simulink subsystem "RoboRio_Controls_sub"  (R2023b)
settings: Solver=VariableStepAuto  StartTime=0.0  StopTime=10.0  RelTol=1e-3
undefined symbols (not defined in the file): Climber_DutyCycle_Neg, Climber_DutyCycle_Pos, Odometry_IC_X, Odometry_IC_Y
libraries: simulink x3, Autonomous_lib x1, Disabled_lib x1, Teleop_lib x1, Test_lib x1
(part 2 of 2)

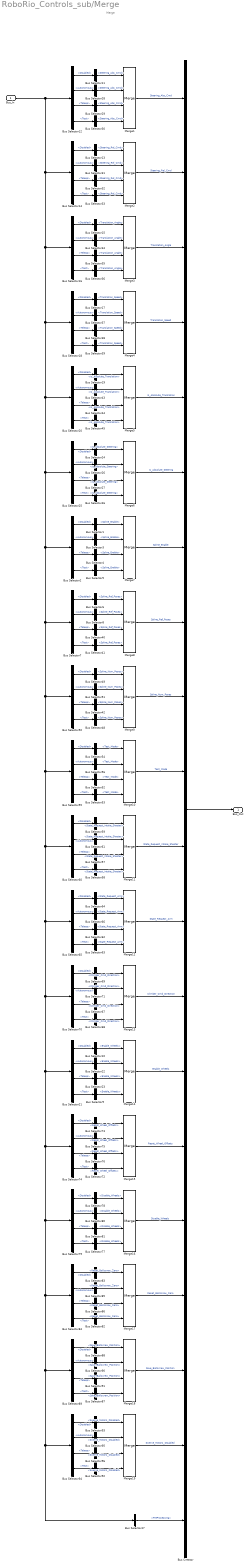
== system RoboRio_Controls_sub/Merge ==
  note: Merge
  Bus_In : Inport
  Bus Creator : BusCreator  Inputs=20
  Bus Selector{1,3..5} (4 alike) : BusSelector  OutputSignals=Spline_Enable
  Bus Selector{9..10,22..23} (4 alike) : BusSelector  OutputSignals=Enable_Wheels
  Bus Selector{11,28..30} (4 alike) : BusSelector  OutputSignals=Steering_Abs_Cmd
  Bus Selector{2,7,12,14,16,18,20..21,25,50,55,60,65,70,74,79,84,89,94} (19 alike) : BusSelector  OutputSignals=Disabled,Autonomous,Teleop,Test
  Bus Selector{13,31..33} (4 alike) : BusSelector  OutputSignals=Steering_Rel_Cmd
  Bus Selector{15,34..36} (4 alike) : BusSelector  OutputSignals=Translation_Angle
  Bus Selector{17,37..39} (4 alike) : BusSelector  OutputSignals=Translation_Speed
  Bus Selector{19,43..45} (4 alike) : BusSelector  OutputSignals=Is_Absolute_Translation
  Bus Selector{24,26..27,46} (4 alike) : BusSelector  OutputSignals=Is_Absolute_Steering
  Bus Selector{6,8,40..41} (4 alike) : BusSelector  OutputSignals=Spline_Ref_Poses
  Bus Selector{42,48..49,51} (4 alike) : BusSelector  OutputSignals=Spline_Num_Poses
  Bus Selector47 : BusSelector  OutputSignals=PreProcessing
  Bus Selector{52..54,56} (4 alike) : BusSelector  OutputSignals=Test_Mode
  Bus Selector{57..59,61} (4 alike) : BusSelector  OutputSignals=State_Request_Intake_Shooter
  Bus Selector{62..64,66} (4 alike) : BusSelector  OutputSignals=State_Request_Arm
  Bus Selector{67..69,71} (4 alike) : BusSelector  OutputSignals=Climber_Cmd_Direction
  Bus Selector{72..73,75..76} (4 alike) : BusSelector  OutputSignals=Reset_Wheel_Offsets
  Bus Selector{77..78,80..81} (4 alike) : BusSelector  OutputSignals=Disable_Wheels
  Bus Selector{82..83,85..86} (4 alike) : BusSelector  OutputSignals=Reset_Ballscrew_Zero
  Bus Selector{87..88,90..91} (4 alike) : BusSelector  OutputSignals=Save_Ballscrew_Position
  Bus Selector{92..93,95..96} (4 alike) : BusSelector  OutputSignals=Swerve_Motors_Disabled
  Merge{1..19} (19 alike) : Merge  Inputs=4
  Bus_Out : Outport
  wires:
  Bus Creator/1 -> Bus_Out/1
  Merge14/1 -> Bus Creator/14  "Enable_Wheels"
  Bus Selector21/4 -> Bus Selector9/1  "<Test>"
  Bus Selector9/1 -> Merge14/4  "<Enable_Wheels>"
  Bus Selector21/3 -> Bus Selector23/1  "<Teleop>"
  Bus Selector21/2 -> Bus Selector22/1  "<Autonomous>"
  Bus Selector10/1 -> Merge14/1  "<Enable_Wheels>"
  Bus_In/1 -> Bus Selector12/1, Bus Selector14/1, Bus Selector16/1, Bus Selector18/1, Bus Selector20/1, Bus Selector25/1, Bus Selector60/1, Bus Selector21/1, Bus Selector74/1, Bus Selector79/1, Bus Selector84/1, Bus Selector89/1, Bus Selector94/1, Bus Selector47/1, Bus Selector70/1, Bus Selector65/1, Bus Selector55/1, Bus Selector50/1, Bus Selector7/1, Bus Selector2/1
  Bus Selector22/1 -> Merge14/2  "<Enable_Wheels>"
  Bus Selector21/1 -> Bus Selector10/1  "<Disabled>"
  Bus Selector23/1 -> Merge14/3  "<Enable_Wheels>"
  Bus Selector94/4 -> Bus Selector92/1  "<Test>"
  Bus Selector93/1 -> Merge19/1  "<Swerve_Motors_Disabled>"
  Bus Selector94/2 -> Bus Selector95/1  "<Autonomous>"
  Bus Selector92/1 -> Merge19/4  "<Swerve_Motors_Disabled>"
  Bus Selector94/3 -> Bus Selector96/1  "<Teleop>"
  Bus Selector94/1 -> Bus Selector93/1  "<Disabled>"
  Bus Selector96/1 -> Merge19/3  "<Swerve_Motors_Disabled>"
  Bus Selector95/1 -> Merge19/2  "<Swerve_Motors_Disabled>"
  Merge19/1 -> Bus Creator/19  "Swerve_Motors_Disabled"
  Merge18/1 -> Bus Creator/18  "Save_Ballscrew_Position"
  Bus Selector89/4 -> Bus Selector87/1  "<Test>"
  Bus Selector88/1 -> Merge18/1  "<Save_Ballscrew_Position>"
  Bus Selector91/1 -> Merge18/3  "<Save_Ballscrew_Position>"
  Bus Selector89/3 -> Bus Selector91/1  "<Teleop>"
  Bus Selector89/2 -> Bus Selector90/1  "<Autonomous>"
  Bus Selector89/1 -> Bus Selector88/1  "<Disabled>"
  Bus Selector87/1 -> Merge18/4  "<Save_Ballscrew_Position>"
  Bus Selector90/1 -> Merge18/2  "<Save_Ballscrew_Position>"
  Bus Selector84/3 -> Bus Selector86/1  "<Teleop>"
  Bus Selector85/1 -> Merge17/2  "<Reset_Ballscrew_Zero>"
  Merge17/1 -> Bus Creator/17  "Reset_Ballscrew_Zero"
  Bus Selector82/1 -> Merge17/4  "<Reset_Ballscrew_Zero>"
  Bus Selector84/4 -> Bus Selector82/1  "<Test>"
  Bus Selector84/2 -> Bus Selector85/1  "<Autonomous>"
  Bus Selector83/1 -> Merge17/1  "<Reset_Ballscrew_Zero>"
  Bus Selector86/1 -> Merge17/3  "<Reset_Ballscrew_Zero>"
  Bus Selector84/1 -> Bus Selector83/1  "<Disabled>"
  Merge16/1 -> Bus Creator/16  "Disable_Wheels"
  Bus Selector81/1 -> Merge16/3  "<Disable_Wheels>"
  Bus Selector79/4 -> Bus Selector77/1  "<Test>"
  Bus Selector79/1 -> Bus Selector78/1  "<Disabled>"
  Bus Selector79/3 -> Bus Selector81/1  "<Teleop>"
  Bus Selector79/2 -> Bus Selector80/1  "<Autonomous>"
  Bus Selector77/1 -> Merge16/4  "<Disable_Wheels>"
  Bus Selector78/1 -> Merge16/1  "<Disable_Wheels>"
  Bus Selector80/1 -> Merge16/2  "<Disable_Wheels>"
  Merge15/1 -> Bus Creator/15  "Reset_Wheel_Offsets"
  Bus Selector74/4 -> Bus Selector72/1  "<Test>"
  Bus Selector74/2 -> Bus Selector75/1  "<Autonomous>"
  Bus Selector74/1 -> Bus Selector73/1  "<Disabled>"
  Bus Selector75/1 -> Merge15/2  "<Reset_Wheel_Offsets>"
  Bus Selector76/1 -> Merge15/3  "<Reset_Wheel_Offsets>"
  Bus Selector74/3 -> Bus Selector76/1  "<Teleop>"
  Bus Selector72/1 -> Merge15/4  "<Reset_Wheel_Offsets>"
  Bus Selector73/1 -> Merge15/1  "<Reset_Wheel_Offsets>"
  Merge13/1 -> Bus Creator/13  "Climber_Cmd_Direction"
  Bus Selector70/3 -> Bus Selector67/1  "<Teleop>"
  Bus Selector67/1 -> Merge13/3  "<Climber_Cmd_Direction>"
  Bus Selector71/1 -> Merge13/2  "<Climber_Cmd_Direction>"
  Bus Selector70/4 -> Bus Selector68/1  "<Test>"
  Bus Selector70/1 -> Bus Selector69/1  "<Disabled>"
  Bus Selector69/1 -> Merge13/1  "<Climber_Cmd_Direction>"
  Bus Selector68/1 -> Merge13/4  "<Climber_Cmd_Direction>"
  Bus Selector70/2 -> Bus Selector71/1  "<Autonomous>"
  Merge12/1 -> Bus Creator/12  "State_Request_Arm"
  Bus Selector65/2 -> Bus Selector66/1  "<Autonomous>"
  Bus Selector63/1 -> Merge12/4  "<State_Request_Arm>"
  Bus Selector64/1 -> Merge12/1  "<State_Request_Arm>"
  Bus Selector65/1 -> Bus Selector64/1  "<Disabled>"
  Bus Selector65/4 -> Bus Selector63/1  "<Test>"
  Bus Selector66/1 -> Merge12/2  "<State_Request_Arm>"
  Bus Selector62/1 -> Merge12/3  "<State_Request_Arm>"
  Bus Selector65/3 -> Bus Selector62/1  "<Teleop>"
  Merge11/1 -> Bus Creator/11  "State_Request_Intake_Shooter"
  Bus Selector60/3 -> Bus Selector57/1  "<Teleop>"
  Bus Selector57/1 -> Merge11/3  "<State_Request_Intake_Shooter>"
  Bus Selector61/1 -> Merge11/2  "<State_Request_Intake_Shooter>"
  Bus Selector60/4 -> Bus Selector58/1  "<Test>"
  Bus Selector60/1 -> Bus Selector59/1  "<Disabled>"
  Bus Selector59/1 -> Merge11/1  "<State_Request_Intake_Shooter>"
  Bus Selector58/1 -> Merge11/4  "<State_Request_Intake_Shooter>"
  Bus Selector60/2 -> Bus Selector61/1  "<Autonomous>"
  Merge10/1 -> Bus Creator/10  "Test_Mode"
  Bus Selector55/2 -> Bus Selector56/1  "<Autonomous>"
  Bus Selector53/1 -> Merge10/4  "<Test_Mode>"
  Bus Selector54/1 -> Merge10/1  "<Test_Mode>"
  Bus Selector55/1 -> Bus Selector54/1  "<Disabled>"
  Bus Selector55/4 -> Bus Selector53/1  "<Test>"
  Bus Selector56/1 -> Merge10/2  "<Test_Mode>"
  Bus Selector52/1 -> Merge10/3  "<Test_Mode>"
  Bus Selector55/3 -> Bus Selector52/1  "<Teleop>"
  Merge9/1 -> Bus Creator/9  "Spline_Num_Poses"
  Bus Selector48/1 -> Merge9/4  "<Spline_Num_Poses>"
  Bus Selector50/1 -> Bus Selector49/1  "<Disabled>"
  Bus Selector42/1 -> Merge9/3  "<Spline_Num_Poses>"
  Bus Selector49/1 -> Merge9/1  "<Spline_Num_Poses>"
  Bus Selector51/1 -> Merge9/2  "<Spline_Num_Poses>"
  Bus Selector50/4 -> Bus Selector48/1  "<Test>"
  Bus Selector50/3 -> Bus Selector42/1  "<Teleop>"
  Bus Selector50/2 -> Bus Selector51/1  "<Autonomous>"
  Merge8/1 -> Bus Creator/8  "Spline_Ref_Poses"
  Bus Selector7/2 -> Bus Selector8/1  "<Autonomous>"
  Bus Selector7/3 -> Bus Selector40/1  "<Teleop>"
  Bus Selector7/4 -> Bus Selector41/1  "<Test>"
  Bus Selector8/1 -> Merge8/2  "<Spline_Ref_Poses>"
  Bus Selector6/1 -> Merge8/1  "<Spline_Ref_Poses>"
  Bus Selector40/1 -> Merge8/3  "<Spline_Ref_Poses>"
  Bus Selector7/1 -> Bus Selector6/1  "<Disabled>"
  Bus Selector41/1 -> Merge8/4  "<Spline_Ref_Poses>"
  Merge7/1 -> Bus Creator/7  "Spline_Enable"
  Bus Selector5/1 -> Merge7/4  "<Spline_Enable>"
  Bus Selector2/1 -> Bus Selector1/1  "<Disabled>"
  Bus Selector4/1 -> Merge7/3  "<Spline_Enable>"
  Bus Selector1/1 -> Merge7/1  "<Spline_Enable>"
  Bus Selector3/1 -> Merge7/2  "<Spline_Enable>"
  Bus Selector2/4 -> Bus Selector5/1  "<Test>"
  Bus Selector2/3 -> Bus Selector4/1  "<Teleop>"
  Bus Selector2/2 -> Bus Selector3/1  "<Autonomous>"
  Bus Selector29/1 -> Merge1/3  "<Steering_Abs_Cmd>"
  Bus Selector25/2 -> Bus Selector26/1  "<Autonomous>"
  Bus Selector25/3 -> Bus Selector27/1  "<Teleop>"
  Bus Selector14/3 -> Bus Selector32/1  "<Teleop>"
  Bus Selector16/3 -> Bus Selector35/1  "<Teleop>"
  Bus Selector16/4 -> Bus Selector36/1  "<Test>"
  Bus Selector20/1 -> Bus Selector19/1  "<Disabled>"
  Merge1/1 -> Bus Creator/1  "Steering_Abs_Cmd"
  Bus Selector34/1 -> Merge3/2  "<Translation_Angle>"
  Bus Selector17/1 -> Merge4/1  "<Translation_Speed>"
  Bus Selector15/1 -> Merge3/1  "<Translation_Angle>"
  Bus Selector20/2 -> Bus Selector43/1  "<Autonomous>"
  Bus Selector14/1 -> Bus Selector13/1  "<Disabled>"
  Bus Selector20/4 -> Bus Selector45/1  "<Test>"
  Merge5/1 -> Bus Creator/5  "Is_Absolute_Translation"
  Bus Selector36/1 -> Merge3/4  "<Translation_Angle>"
  Bus Selector47/1 -> Bus Creator/20  "<PreProcessing>"
  Bus Selector12/1 -> Bus Selector11/1  "<Disabled>"
  Bus Selector16/2 -> Bus Selector34/1  "<Autonomous>"
  Bus Selector37/1 -> Merge4/2  "<Translation_Speed>"
  Bus Selector25/4 -> Bus Selector46/1  "<Test>"
  Bus Selector18/3 -> Bus Selector38/1  "<Teleop>"
  Bus Selector20/3 -> Bus Selector44/1  "<Teleop>"
  Bus Selector39/1 -> Merge4/4  "<Translation_Speed>"
  Bus Selector16/1 -> Bus Selector15/1  "<Disabled>"
  Bus Selector13/1 -> Merge2/1  "<Steering_Rel_Cmd>"
  Bus Selector30/1 -> Merge1/4  "<Steering_Abs_Cmd>"
  Bus Selector26/1 -> Merge6/2  "<Is_Absolute_Steering>"
  Merge6/1 -> Bus Creator/6  "Is_Absolute_Steering"
  Bus Selector18/1 -> Bus Selector17/1  "<Disabled>"
  Bus Selector45/1 -> Merge5/4  "<Is_Absolute_Translation>"
  Bus Selector12/3 -> Bus Selector29/1  "<Teleop>"
  Bus Selector18/2 -> Bus Selector37/1  "<Autonomous>"
  Bus Selector43/1 -> Merge5/2  "<Is_Absolute_Translation>"
  Bus Selector19/1 -> Merge5/1  "<Is_Absolute_Translation>"
  Bus Selector35/1 -> Merge3/3  "<Translation_Angle>"
  Merge3/1 -> Bus Creator/3  "Translation_Angle"
  Bus Selector28/1 -> Merge1/2  "<Steering_Abs_Cmd>"
  Bus Selector14/2 -> Bus Selector31/1  "<Autonomous>"
  Bus Selector32/1 -> Merge2/3  "<Steering_Rel_Cmd>"
  Merge4/1 -> Bus Creator/4  "Translation_Speed"
  Bus Selector12/2 -> Bus Selector28/1  "<Autonomous>"
  Bus Selector14/4 -> Bus Selector33/1  "<Test>"
  Bus Selector44/1 -> Merge5/3  "<Is_Absolute_Translation>"
  Bus Selector24/1 -> Merge6/1  "<Is_Absolute_Steering>"
  Bus Selector11/1 -> Merge1/1  "<Steering_Abs_Cmd>"
  Bus Selector31/1 -> Merge2/2  "<Steering_Rel_Cmd>"
  Bus Selector27/1 -> Merge6/3  "<Is_Absolute_Steering>"
  Bus Selector25/1 -> Bus Selector24/1  "<Disabled>"
  Bus Selector18/4 -> Bus Selector39/1  "<Test>"
  Bus Selector46/1 -> Merge6/4  "<Is_Absolute_Steering>"
  Bus Selector38/1 -> Merge4/3  "<Translation_Speed>"
  Bus Selector33/1 -> Merge2/4  "<Steering_Rel_Cmd>"
  Bus Selector12/4 -> Bus Selector30/1  "<Test>"
  Merge2/1 -> Bus Creator/2  "Steering_Rel_Cmd"

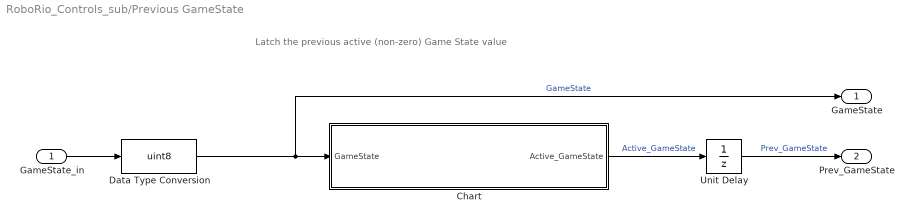
== system RoboRio_Controls_sub/Previous GameState ==
  note: Latch the previous active (non-zero) Game State value
  GameState_in : Inport
  Chart : Stateflow chart  TreatAsAtomicUnit=on
  Data Type Conversion : DataTypeConversion  OutDataTypeStr=uint8  SaturateOnIntegerOverflow=off  RndMeth=Floor
  Unit Delay : UnitDelay  SampleTime=-1  HasFrameUpgradeWarning=on
  GameState : Outport
  Prev_GameState : Outport  Port=2
  wires:
  Chart/1(Active_GameState) -> Unit Delay/1  "Active_GameState"
  Data Type Conversion/1 -> Chart/1(GameState), GameState/1  "GameState"
  Unit Delay/1 -> Prev_GameState/1  "Prev_GameState"
  GameState_in/1 -> Data Type Conversion/1

== stateflow chart RoboRio_Controls_sub/Previous GameState/Chart ==
  state Disabled
  state Not_Disabled
    en: Active_GameState = GameState;
    du: Active_GameState = GameState;
  (default) -> Disabled : {Active_GameState = 0}
  Disabled -> Not_Disabled : [GameState ~= 0]
  Not_Disabled -> Disabled : [GameState == 0]
  data: GameState input; Active_GameState output
